simulink model "Model_6DOF_B3"  (R2020b)
settings: Solver=FixedStepAuto  StartTime=0.0  StopTime=120  FixedStep=0.05  RelTol=1e-3
values from neighbouring files (symbols this model uses):
  Ba_0 = [0 0 0 0 0 0]    [ctrl_mode_param.m]
  Bb = 4418825.3321    [load_data.m]
  Bv_0 = [tgt_speed 0 0 0 0 0]    [ctrl_mode_param.m]
  Bx_0 = [0 0 tgt_depth 0 0 0]    [ctrl_mode_param.m]
  Ixx = 5.23e7    (= 52300000)    [load_data.m]
  Ixy = 0    [load_data.m]
  Ixz = 0    [load_data.m]
  Iyy = 1.375e9    (= 1375000000)    [load_data.m]
  Iyz = 0    [load_data.m]
  Izz = 1.367e9    (= 1367000000)    [load_data.m]
  Mb = 4418825.3321    [load_data.m]
  Xb = 0    [load_data.m]
  Xg = 0    [load_data.m]
  Yb = 0    [load_data.m]
  Yg = 0    [load_data.m]
  Zb = 0.4406    [load_data.m]
  Zg = 0    [load_data.m]
undefined symbols (not defined in the file or in its folder): dA_BP1, dA_BP2, dA_Hull, dA_PH, dA_Sail, dA_SProot, dA_X1a, dA_X1b, dA_X2a, dA_X2b, dA_X3a, dA_X3b, dA_X4a, dA_X4b, its, n_BP1, n_BP2, n_Hull, n_PH, n_Sail, n_SProot, n_X1a, n_X1b, n_X2a, n_X2b, n_X3a, n_X3b, n_X4a, n_X4b, nt_BP1, nt_BP2, nt_Hull, nt_PH, nt_Sail, nt_SProot, nt_X1a, nt_X1b, nt_X2a, nt_X2b, nt_X3a, nt_X3b, nt_X4a, nt_X4b, Usp, vt1_BP1, vt1_BP2, vt1_Hull, vt1_PH, vt1_Sail, vt1_SProot, vt1_X1a, vt1_X1b, vt1_X2a, vt1_X2b, vt1_X3a, vt1_X3b, vt1_X4a, vt1_X4b, vt2_BP1, vt2_BP2 ... (+27)
libraries: simulink x5
(part 9 of 15)

== system Model_6DOF_B3/HDM B3/Wave, Virtual Mass and Hydrostatic/Wave Particle Motions ==
  U_ship : Inport
  X_earth : Inport  Port=2
  CGi : Inport  Port=3
  CG : Inport  Port=4
  SeaState : Inport  Port=5
  dLCG : Inport  Port=6
  dX_CTRL : Inport  Port=7
  fwrite : Inport  Port=8
  Add : Sum  Inputs=+-
  Clock : Clock
  Constant : Constant  Value=3
  Constant1 : Constant  Value=Zb
  Constant2 : Constant  Value=0.474
  Constant6 : Constant  Value=1025
  Constant7 : Constant  Value=9.81
  Local eff. Depth : MATLAB Function  TreatAsAtomicUnit=on
  MATLAB Function1 : MATLAB Function  TreatAsAtomicUnit=on
  Mux : Mux  Inputs=5
  Sectional Position Vectors : MATLAB Function  TreatAsAtomicUnit=on
  Sectional Wave Particle & Rigid Body Velocities : MATLAB Function  TreatAsAtomicUnit=on
  Subsystem : Subsystem
  Wave Properties : MATLAB Function  TreatAsAtomicUnit=on
  Wave particle velocity at hull CG : MATLAB Function  TreatAsAtomicUnit=on
  X_SP1 : Constant  Value=[31.924; 3.861; -3.861;]
  X_SP2 : Constant  Value=[31.924; 3.861; 3.861;]
  X_SP3 : Constant  Value=[31.924; -3.861; 3.861;]
  X_SP4 : Constant  Value=[31.924; -3.861; -3.861;]
  X_XB : Constant  Value=[-10.465; 0; 9.732;]
  beta_wave : Constant  Value=0
  phi_wave : Constant  Value=0
  Rs : Outport
  zeff : Outport  Port=2
  uwXis : Outport  Port=3
  uwsCG : Outport  Port=4
  uws : Outport  Port=5
  urs : Outport  Port=6
  B_FM : Outport  Port=7
  wires:
  Sectional Position Vectors/2(Rs) -> Sectional Wave Particle & Rigid Body Velocities/5(Rs), Rs/1
  SeaState/1 -> Wave Properties/1(SeaState)
  Clock/1 -> MATLAB Function1/1(time), Wave particle velocity at hull CG/1(time), Local eff. Depth/1(time), Sectional Wave Particle & Rigid Body Velocities/1(time), Subsystem/1(time)
  Sectional Position Vectors/1(Xce) -> Sectional Wave Particle & Rigid Body Velocities/4(Xce)
  X_earth/1 -> Subsystem/2(Xearth), Sectional Wave Particle & Rigid Body Velocities/3(X_earth), MATLAB Function1/7(X_earth), Wave particle velocity at hull CG/2(X_earth), Local eff. Depth/2(Bxe), Sectional Position Vectors/1(X_earth)
  Wave Properties/3(k_wave) -> Subsystem/4(k_wave), Wave particle velocity at hull CG/8(k_wave), Local eff. Depth/3(k_wave), MATLAB Function1/13(k_wave), Sectional Wave Particle & Rigid Body Velocities/10(k_wave)  "k"
  U_ship/1 -> MATLAB Function1/8(U_ship), Sectional Wave Particle & Rigid Body Velocities/2(U_ship)
  Wave Properties/1(L_wave) -> MATLAB Function1/9(L_wave), Sectional Wave Particle & Rigid Body Velocities/8(L_wave), Wave particle velocity at hull CG/4(L_wave)
  Wave Properties/4(w_wave) -> Subsystem/5(w_wave), Wave particle velocity at hull CG/9(w_wave), Local eff. Depth/4(w_wave), MATLAB Function1/14(w_wave), Sectional Wave Particle & Rigid Body Velocities/11(w_wave)  "w"
  CGi/1 -> Sectional Position Vectors/2(CGi)
  CG/1 -> Sectional Position Vectors/3(CG)
  Sectional Wave Particle & Rigid Body Velocities/2(Urs) -> urs/1
  Sectional Wave Particle & Rigid Body Velocities/1(Uws) -> uws/1
  dLCG/1 -> Wave particle velocity at hull CG/3(dLCG), Sectional Position Vectors/4(dLCG)
  Wave Properties/2(A_wave) -> Subsystem/3(A_wave), Wave particle velocity at hull CG/7(A_wave), Local eff. Depth/5(a_wave), MATLAB Function1/12(A_wave), Sectional Wave Particle & Rigid Body Velocities/9(A_wave)
  Local eff. Depth/1(z_eff) -> zeff/1
  X_XB/1 -> MATLAB Function1/6(rXB)
  X_SP4/1 -> MATLAB Function1/5(rX4)
  X_SP3/1 -> MATLAB Function1/4(rX3)
  X_SP2/1 -> MATLAB Function1/3(rX2)
  X_SP1/1 -> MATLAB Function1/2(rX1)
  MATLAB Function1/1(uwX1s) -> Mux/1
  MATLAB Function1/2(uwX2s) -> Mux/2
  MATLAB Function1/3(uwX3s) -> Mux/3
  MATLAB Function1/4(uwX4s) -> Mux/4
  MATLAB Function1/5(uwXBs) -> Mux/5
  Mux/1 -> uwXis/1
  phi_wave/1 -> Sectional Wave Particle & Rigid Body Velocities/6(phi_wave), Wave particle velocity at hull CG/5(phi_wave), MATLAB Function1/10(phi_wave)
  beta_wave/1 -> MATLAB Function1/11(beta_wave), Sectional Wave Particle & Rigid Body Velocities/7(beta_wave), Wave particle velocity at hull CG/6(beta_wave)
  Wave particle velocity at hull CG/1(uwsCG) -> uwsCG/1
  Constant/1 -> Sectional Wave Particle & Rigid Body Velocities/12(iProbe)
  Subsystem/1(Out1) -> B_FM/1
  Constant6/1 -> Subsystem/6(rho)
  Constant7/1 -> Subsystem/7(g)
  Add/1 -> Subsystem/8(Zb)
  Constant2/1 -> Add/1
  Constant1/1 -> Add/2
  dX_CTRL/1 -> Subsystem/9(dX_CTRL)
  fwrite/1 -> Subsystem/10(fwrite)

== system Model_6DOF_B3/HDM B3/X/X'dXi ==
  UeX : Inport
  dXeff : Inport  Port=2
  Gain : Gain  Gain=-1
  Gain{4..7} (4 alike) : Gain
  Mux : Mux  Inputs=5
  Saturation6 : Saturate  UpperLimit=-1.543332  LowerLimit=-5.14444
  Selector10 : Selector  InputPortWidth=5  IndexOptions=Index vector (dialog)  Indices=4  OutputSizes=1
  Selector11 : Selector  InputPortWidth=5  IndexOptions=Index vector (dialog)  Indices=4  OutputSizes=1
  Selector12 : Selector  InputPortWidth=5  IndexOptions=Index vector (dialog)  Indices=5  OutputSizes=1
  Selector2 : Selector  InputPortWidth=5  IndexOptions=Index vector (dialog)  Indices=5  OutputSizes=1
  Selector4 : Selector  InputPortWidth=5  IndexOptions=Index vector (dialog)  Indices=1  OutputSizes=1
  Selector5 : Selector  InputPortWidth=5  IndexOptions=Index vector (dialog)  Indices=1  OutputSizes=1
  Selector6 : Selector  InputPortWidth=5  IndexOptions=Index vector (dialog)  Indices=2  OutputSizes=1
  Selector7 : Selector  InputPortWidth=5  IndexOptions=Index vector (dialog)  Indices=2  OutputSizes=1
  Selector8 : Selector  InputPortWidth=5  IndexOptions=Index vector (dialog)  Indices=3  OutputSizes=1
  Selector9 : Selector  InputPortWidth=5  IndexOptions=Index vector (dialog)  Indices=3  OutputSizes=1
  To Workspace : ToWorkspace  VariableName=UeX  SaveFormat=Timeseries  SampleTime=-1
  XudX1 : Lookup_n-D  BreakpointsForDimension1=[-30 -20 -10 0 10 20 30]  BreakpointsForDimension2=|  Table=|  InternalRulePriority=Speed  RndMeth=Simplest  InputSameDT=on
      BreakpointsForDimension2=|
      | [-7.716666
      | -5.144444
      | -3.0866664
      | -1.5433332
      | ]
      Table=|
      | reshape([3.2151E-04
      | 1.4055E-04
      | 2.3723E-05
      | -2.9685E-05
      | 2.3777E-05
      | 1.3375E-04
      | 3.3722E-04
      | 1.6076E-04
      | 7.0275E-05
      | 1.1862E-05
      | -1.4843E-05
      | 1.1889E-05
      | 6.6875E-05
      | 1.6861E-04
      | 1.6698E-04
      | 6.8790E-05
      | 1.2322E-05
      | -1.4312E-05
      | 1.2274E-05
      | 6.7265E-05
      | 1.7083E-04
      | 3.4224E-04
      | 1.3333E-04
      | 2.5937E-05
      | -6.5668E-05
      | 2.5937E-05
      | 1.3102E-04
      | 3.4214E-04
      | ],[7,4])
      settings: InputPortMap=u0,u1
  XudX2 : Lookup_n-D  BreakpointsForDimension1=[-30 -20 -10 0 10 20 30]  BreakpointsForDimension2=|  Table=|  InternalRulePriority=Speed  RndMeth=Simplest  InputSameDT=on
      BreakpointsForDimension2=|
      | [-7.716666
      | -5.144444
      | -3.0866664
      | -1.5433332
      | ]
      Table=|
      | reshape([2.9233E-04
      | 1.3189E-04
      | 2.3224E-05
      | -2.9022E-05
      | 1.9675E-05
      | 1.4726E-04
      | 3.7676E-04
      | 1.4617E-04
      | 6.5945E-05
      | 1.1612E-05
      | -1.4511E-05
      | 9.8375E-06
      | 7.3630E-05
      | 1.8838E-04
      | 1.7319E-04
      | 6.7285E-05
      | 1.2060E-05
      | -2.5958E-05
      | 1.0337E-05
      | 7.6660E-05
      | 1.8963E-04
      | 3.4748E-04
      | 1.3335E-04
      | 2.2395E-05
      | -2.6403E-05
      | 2.2395E-05
      | 1.5181E-04
      | 3.8598E-04
      | ],[7,4])
      settings: InputPortMap=u0,u1
  XudX3 : Lookup_n-D  BreakpointsForDimension1=[-30 -20 -10 0 10 20 30]  BreakpointsForDimension2=|  Table=|  InternalRulePriority=Speed  RndMeth=Simplest  InputSameDT=on
      BreakpointsForDimension2=|
      | [-7.716666
      | -5.144444
      | -3.0866664
      | -1.5433332
      | ]
      Table=|
      | reshape([3.5642E-04
      | 1.5674E-04
      | 2.5449E-05
      | -2.9060E-05
      | 2.6726E-05
      | 1.6225E-04
      | 3.1115E-04
      | 1.7821E-04
      | 7.8370E-05
      | 1.2725E-05
      | -1.4530E-05
      | 1.3363E-05
      | 8.1125E-05
      | 1.5558E-04
      | 1.9053E-04
      | 8.0600E-05
      | 1.2911E-05
      | -1.3998E-05
      | 1.3672E-05
      | 7.4645E-05
      | 1.6290E-04
      | 3.8447E-04
      | 1.4526E-04
      | 2.7824E-05
      | -2.6434E-05
      | 2.7824E-05
      | 1.5039E-04
      | 3.2499E-04
      | ],[7,4])
      settings: InputPortMap=u0,u1
  XudX4 : Lookup_n-D  BreakpointsForDimension1=[-30 -20 -10 0 10 20 30]  BreakpointsForDimension2=|  Table=|  InternalRulePriority=Speed  RndMeth=Simplest  InputSameDT=on
      BreakpointsForDimension2=|
      | [-7.716666
      | -5.144444
      | -3.0866664
      | -1.5433332
      | ]
      Table=|
      | reshape([3.4525E-04
      | 1.3840E-04
      | 2.4668E-05
      | -2.9702E-05
      | 2.4205E-05
      | 1.2737E-04
      | 3.2790E-04
      | 1.7263E-04
      | 6.9200E-05
      | 1.2334E-05
      | -1.4851E-05
      | 1.2103E-05
      | 6.3685E-05
      | 1.6395E-04
      | 1.7298E-04
      | 6.9435E-05
      | 1.2696E-05
      | -1.4315E-05
      | 1.2608E-05
      | 6.9175E-05
      | 1.6779E-04
      | 3.3803E-04
      | 1.5513E-04
      | 2.6677E-05
      | -2.7052E-05
      | 2.6677E-05
      | 1.3644E-04
      | 3.3780E-04
      | ],[7,4])
      settings: InputPortMap=u0,u1
  XudXB : Lookup_n-D  BreakpointsForDimension1=[-30 -20 -10 0 10 20 30]  BreakpointsForDimension2=[-5.14444 -3.08666664 -1.54332]  Table=|  InternalRulePriority=Speed  RndMeth=Simplest  InputSameDT=on
      | reshape([6.9060E-04
      | 3.9256E-04
      | 1.5651E-04
      | 0.0000E+00
      | 1.1449E-04
      | 4.2412E-04
      | 5.7370E-04
      | 6.4542E-04
      | 3.9138E-04
      | 1.5593E-04
      | 0.0000E+00
      | 1.1381E-04
      | 4.1205E-04
      | 5.6813E-04
      | 6.5675E-04
      | 3.9410E-04
      | 1.1271E-04
      | 0.0000E+00
      | 1.1271E-04
      | 4.2649E-04
      | 5.7604E-04
      | ],[7,3])
      settings: InputPortMap=u0,u1
  Out1 : Outport
  wires:
  Selector2/1 -> XudXB/1
  XudX4/1 -> Gain7/1
  XudX3/1 -> Gain5/1
  XudX2/1 -> Gain6/1
  XudX1/1 -> Gain4/1
  Mux/1 -> Out1/1
  dXeff/1 -> Selector2/1, Selector10/1, Selector8/1, Selector6/1, Selector4/1
  Selector4/1 -> XudX1/1
  Selector5/1 -> XudX1/2
  Selector6/1 -> XudX2/1
  Selector7/1 -> XudX2/2
  Selector8/1 -> XudX3/1
  Selector9/1 -> XudX3/2
  UeX/1 -> Gain/1
  Selector11/1 -> XudX4/2
  Selector10/1 -> XudX4/1
  Selector12/1 -> XudXB/2
  Gain4/1 -> Mux/1
  Gain6/1 -> Mux/2
  Gain5/1 -> Mux/3
  Gain7/1 -> Mux/4
  XudXB/1 -> Mux/5
  Gain/1 -> To Workspace/1, Saturation6/1
  Saturation6/1 -> Selector11/1, Selector12/1, Selector9/1, Selector7/1, Selector5/1

== system Model_6DOF_B3/HDM B3/X 6d org/Subsystem1 ==
  UeX : Inport
  dXeff : Inport  Port=2
  z : Inport  Port=3
  Demux : Demux  Outputs=5
  Demux1 : Demux  Outputs=5
  Mux : Mux  Inputs=5
  Xud4 : Lookup_n-D  NumberOfTableDimensions=3  BreakpointsForDimension1=[-30 -20 -10 0 10 20 30]  BreakpointsForDimension2=|  BreakpointsForDimension3=|  Table=|  InternalRulePriority=Speed  RndMeth=Simplest  InputSameDT=on
      BreakpointsForDimension2=|
      | [1.5433332
      | 3.0866664
      | 
      | 5.144444]
      BreakpointsForDimension3=|
      | [-36.3724
      | -18.3724
      | -15.3724
      | -13.8724]
      Table=|
      | reshape([1.9515E-04
      | 1.0370E-04
      | 3.9468E-05
      | 1.2612E-05
      | 3.9477E-05
      | 9.2497E-05
      | 1.9504E-04
      | 2.0037E-04
      | 9.3994E-05
      | 3.9650E-05
      | 1.2608E-05
      | 3.9217E-05
      | 9.5451E-05
      | 1.8893E-04
      | 2.0342E-04
      | 9.8349E-05
      | 3.9739E-05
      | 1.2608E-05
      | 3.9126E-05
      | 9.3002E-05
      | 1.9310E-04
      | 2.0342E-04
      | 9.7784E-05
      | 3.9737E-05
      | 1.2594E-05
      | 3.8955E-05
      | 9.3472E-05
      | 1.8818E-04
      | 1.9912E-04
      | 9.6216E-05
      | 3.8834E-05
      | 1.1823E-05
      | 3.8745E-05
      | 9.5316E-05
      | 1.9299E-04
      | 2.0055E-04
      | 9.7244E-05
      | 3.9050E-05
      | 1.1812E-05
      | 3.8434E-05
      | 9.0497E-05
      | 1.8966E-04
      | 2.6693E-04
      | 1.4022E-04
      | 3.8561E-05
      | 1.1822E-05
      | 3.3455E-05
      | 1.0520E-04
      | 2.4359E-04
      | 2.0044E-04
      | 1.0295E-04
      | 3.9158E-05
      | 1.1774E-05
      | 3.8178E-05
      | 9.0714E-05
      | 1.8818E-04
      | 1.9655E-04
      | 9.5339E-05
      | 3.8472E-05
      | 1.1287E-05
      | 3.8241E-05
      | 9.3683E-05
      | 1.8812E-04
      | 1.9890E-04
      | 9.7584E-05
      | 3.8662E-05
      | 1.1263E-05
      | 3.7865E-05
      | 8.8045E-05
      | 1.8986E-04
      | 2.6693E-04
      | 1.4022E-04
      | 3.8561E-05
      | 1.1263E-05
      | 3.3455E-05
      | 1.0520E-04
      | 2.4359E-04
      | 2.0199E-04
      | 9.6354E-05
      | 3.8835E-05
      | 1.1203E-05
      | 3.7555E-05
      | 8.7551E-05
      | 1.8761E-04],[7,3,4])
      settings: InputPortMap=u0,u1,u2
  XudX1 : Lookup_n-D  NumberOfTableDimensions=3  BreakpointsForDimension1=[-30 -20 -10 0 10 20 30]  BreakpointsForDimension2=|  BreakpointsForDimension3=|  Table=|  InternalRulePriority=Speed  RndMeth=Simplest  InputSameDT=on
      BreakpointsForDimension2=|
      | [1.5433332
      | 3.0866664
      | 
      | 5.144444]
      BreakpointsForDimension3=|
      | [-36.3724
      | -18.3724
      | -15.3724
      | -13.8724]
      Table=|
      | reshape([1.9726E-04
      | 9.2807E-05
      | 3.9153E-05
      | 1.2612E-05
      | 3.9108E-05
      | 9.6157E-05
      | 1.9721E-04
      | 1.9513E-04
      | 9.5505E-05
      | 3.8964E-05
      | 1.2607E-05
      | 3.9329E-05
      | 9.6357E-05
      | 1.9540E-04
      | 1.9473E-04
      | 1.0389E-04
      | 3.8933E-05
      | 1.2607E-05
      | 3.9448E-05
      | 9.9420E-05
      | 2.0231E-04
      | 1.9473E-04
      | 1.0019E-04
      | 3.8828E-05
      | 1.2592E-05
      | 3.9441E-05
      | 9.3211E-05
      | 2.0035E-04
      | 1.9312E-04
      | 9.4955E-05
      | 3.8460E-05
      | 1.1826E-05
      | 3.8411E-05
      | 9.3406E-05
      | 1.9672E-04
      | 1.9062E-04
      | 9.2834E-05
      | 3.8250E-05
      | 1.1814E-05
      | 3.8668E-05
      | 9.2911E-05
      | 1.9753E-04
      | 2.4353E-04
      | 1.0500E-04
      | 3.3326E-05
      | 1.1821E-05
      | 3.8282E-05
      | 1.3081E-04
      | 2.5995E-04
      | 1.8933E-04
      | 9.3556E-05
      | 3.8050E-05
      | 1.1773E-05
      | 3.8871E-05
      | 9.3887E-05
      | 2.0035E-04
      | 1.8690E-04
      | 9.6416E-05
      | 3.7999E-05
      | 1.1295E-05
      | 3.8027E-05
      | 9.1995E-05
      | 1.9449E-04
      | 1.9009E-04
      | 9.2479E-05
      | 3.7675E-05
      | 1.1269E-05
      | 3.8335E-05
      | 8.9889E-05
      | 1.9665E-04
      | 2.4353E-04
      | 1.0500E-04
      | 3.3326E-05
      | 1.1269E-05
      | 3.8282E-05
      | 1.3081E-04
      | 2.5995E-04
      | 1.8646E-04
      | 9.1163E-05
      | 3.7419E-05
      | 1.1206E-05
      | 3.8643E-05
      | 9.8736E-05
      | 2.0514E-04],[7,3,4])
      settings: InputPortMap=u0,u1,u2
  XudX1B : Lookup_n-D  NumberOfTableDimensions=3  BreakpointsForDimension1=[-30 -20 -10 0 10 20 30]  BreakpointsForDimension2=|  BreakpointsForDimension3=|  Table=|  InternalRulePriority=Speed  RndMeth=Simplest  InputSameDT=on
      BreakpointsForDimension2=|
      | [1.5433332
      | 3.0866664
      | 
      | 5.144444]
      BreakpointsForDimension3=|
      | [-36.3724
      | -18.3724
      | -15.3724
      | -13.8724]
      Table=|
      | reshape([3.9535E-04
      | 2.6403E-04
      | 1.4465E-04
      | 6.6976E-05
      | 1.2333E-04
      | 2.8515E-04
      | 3.5499E-04
      | 3.8973E-04
      | 2.6514E-04
      | 1.4731E-04
      | 6.8622E-05
      | 1.2628E-04
      | 2.9201E-04
      | 3.6632E-04
      | 4.0285E-04
      | 2.7250E-04
      | 1.4933E-04
      | 6.8622E-05
      | 1.2952E-04
      | 2.9373E-04
      | 3.6588E-04
      | 4.0285E-04
      | 2.8332E-04
      | 1.5162E-04
      | 7.2213E-05
      | 1.3467E-04
      | 3.0293E-04
      | 3.6349E-04
      | 3.8950E-04
      | 2.6292E-04
      | 1.4475E-04
      | 6.6785E-05
      | 1.2369E-04
      | 2.7281E-04
      | 3.4895E-04
      | 3.9519E-04
      | 2.6529E-04
      | 1.4760E-04
      | 6.8542E-05
      | 1.2717E-04
      | 2.7841E-04
      | 3.6301E-04
      | 5.6904E-04
      | 3.2107E-04
      | 1.3512E-04
      | 7.0542E-05
      | 1.0919E-04
      | 4.1259E-04
      | 6.2735E-04
      | 3.6838E-04
      | 3.0195E-04
      | 1.5438E-04
      | 7.4592E-05
      | 1.4048E-04
      | 3.1396E-04
      | 3.6349E-04
      | 4.1126E-04
      | 2.6224E-04
      | 1.4422E-04
      | 6.5961E-05
      | 1.2321E-04
      | 2.7802E-04
      | 3.5744E-04
      | 4.0057E-04
      | 2.6952E-04
      | 1.4782E-04
      | 6.8341E-05
      | 1.2789E-04
      | 2.8978E-04
      | 3.5944E-04
      | 5.6904E-04
      | 3.2107E-04
      | 1.3512E-04
      | 6.8341E-05
      | 1.0919E-04
      | 4.1259E-04
      | 6.2735E-04
      | 4.8319E-04
      | 3.1751E-04
      | 1.5761E-04
      | 7.4804E-05
      | 1.3557E-04
      | 3.2741E-04
      | 4.7146E-04],[7,3,4])
      settings: InputPortMap=u0,u1,u2
  XudX2 : Lookup_n-D  NumberOfTableDimensions=3  BreakpointsForDimension1=[-30 -20 -10 0 10 20 30]  BreakpointsForDimension2=|  BreakpointsForDimension3=|  Table=|  InternalRulePriority=Speed  RndMeth=Simplest  InputSameDT=on
      BreakpointsForDimension2=|
      | [1.5433332
      | 3.0866664
      | 
      | 5.144444]
      BreakpointsForDimension3=|
      | [-36.3724
      | -18.3724
      | -15.3724
      | -13.8724]
      Table=|
      | reshape([1.9988E-04
      | 9.2815E-05
      | 3.8984E-05
      | 1.2936E-05
      | 3.7333E-05
      | 1.0938E-04
      | 2.1913E-04
      | 2.0000E-04
      | 9.3101E-05
      | 3.8429E-05
      | 1.2739E-05
      | 3.7583E-05
      | 1.1064E-04
      | 2.1950E-04
      | 2.0083E-04
      | 9.4269E-05
      | 3.8054E-05
      | 1.2739E-05
      | 3.7662E-05
      | 1.0858E-04
      | 2.2083E-04
      | 2.0083E-04
      | 9.5605E-05
      | 3.7864E-05
      | 1.2538E-05
      | 3.7776E-05
      | 1.1595E-04
      | 2.1404E-04
      | 1.9933E-04
      | 9.2999E-05
      | 3.8198E-05
      | 1.2159E-05
      | 3.6475E-05
      | 1.0280E-04
      | 2.1737E-04
      | 2.0006E-04
      | 9.3307E-05
      | 3.7549E-05
      | 1.1957E-05
      | 3.6899E-05
      | 1.1530E-04
      | 2.2066E-04
      | 2.4216E-04
      | 1.0448E-04
      | 2.9342E-05
      | 1.1821E-05
      | 3.5012E-05
      | 1.3098E-04
      | 2.3359E-04
      | 1.9082E-04
      | 9.0828E-05
      | 3.6826E-05
      | 1.1709E-05
      | 3.7301E-05
      | 1.0927E-04
      | 2.1404E-04
      | 1.6701E-04
      | 9.2083E-05
      | 3.7750E-05
      | 1.1627E-05
      | 3.5975E-05
      | 9.9381E-05
      | 2.1803E-04
      | 1.9264E-04
      | 9.0003E-05
      | 3.6917E-05
      | 1.1397E-05
      | 3.6539E-05
      | 1.0523E-04
      | 2.1540E-04
      | 2.4216E-04
      | 1.0448E-04
      | 2.9342E-05
      | 1.1397E-05
      | 3.5012E-05
      | 1.3098E-04
      | 2.3359E-04
      | 1.8911E-04
      | 9.0019E-05
      | 3.6083E-05
      | 1.1213E-05
      | 3.7708E-05
      | 1.0882E-04
      | 1.6878E-04],[7,3,4])
      settings: InputPortMap=u0,u1,u2
  XudX3 : Lookup_n-D  NumberOfTableDimensions=3  BreakpointsForDimension1=[-30 -20 -10 0 10 20 30]  BreakpointsForDimension2=|  BreakpointsForDimension3=|  Table=|  InternalRulePriority=Speed  RndMeth=Simplest  InputSameDT=on
      BreakpointsForDimension2=|
      | [1.5433332
      | 3.0866664
      | 
      | 5.144444]
      BreakpointsForDimension3=|
      | [-36.3724
      | -18.3724
      | -15.3724
      | -13.8724]
      Table=|
      | reshape([2.1838E-04
      | 9.8768E-05
      | 3.9298E-05
      | 1.2921E-05
      | 4.0048E-05
      | 1.0549E-04
      | 1.8864E-04
      | 2.2881E-04
      | 1.0336E-04
      | 3.9060E-05
      | 1.2736E-05
      | 3.9535E-05
      | 1.0325E-04
      | 1.9538E-04
      | 2.1692E-04
      | 1.0227E-04
      | 3.8885E-05
      | 1.2736E-05
      | 3.9285E-05
      | 9.9666E-05
      | 1.9406E-04
      | 2.1692E-04
      | 1.0151E-04
      | 3.8619E-05
      | 1.2552E-05
      | 3.9212E-05
      | 1.0291E-04
      | 2.0160E-04
      | 2.1667E-04
      | 1.0323E-04
      | 3.9049E-05
      | 1.2140E-05
      | 3.9810E-05
      | 1.0079E-04
      | 1.9039E-04
      | 2.2496E-04
      | 9.9708E-05
      | 3.8786E-05
      | 1.1948E-05
      | 3.9280E-05
      | 1.0040E-04
      | 1.8622E-04
      | 2.7315E-04
      | 1.3714E-04
      | 3.4983E-05
      | 1.1821E-05
      | 3.1018E-05
      | 1.0427E-04
      | 1.9674E-04
      | 2.2211E-04
      | 1.0444E-04
      | 3.8528E-05
      | 1.1713E-05
      | 3.8636E-05
      | 9.5401E-05
      | 2.0160E-04
      | 2.0348E-04
      | 1.0451E-04
      | 3.8863E-05
      | 1.1608E-05
      | 3.9501E-05
      | 1.0479E-04
      | 1.8840E-04
      | 2.0541E-04
      | 9.7216E-05
      | 3.8561E-05
      | 1.1388E-05
      | 3.8824E-05
      | 9.5169E-05
      | 1.8576E-04
      | 2.7315E-04
      | 1.3714E-04
      | 3.4983E-05
      | 1.1388E-05
      | 3.1018E-05
      | 1.0427E-04
      | 1.9674E-04
      | 2.1961E-04
      | 1.1536E-04
      | 3.8716E-05
      | 1.1221E-05
      | 3.7813E-05
      | 9.5976E-05
      | 1.9612E-04],[7,3,4])
      settings: InputPortMap=u0,u1,u2
  XdXi : Outport
  wires:
  Mux/1 -> XdXi/1
  XudX1/1 -> Mux/1
  XudX2/1 -> Mux/2
  Xud4/1 -> Mux/4
  dXeff/1 -> Demux1/1
  UeX/1 -> Demux/1
  XudX3/1 -> Mux/3
  XudX1B/1 -> Mux/5
  Demux/1 -> XudX1/2
  Demux/2 -> XudX2/2
  Demux/3 -> XudX3/2
  Demux/4 -> Xud4/2
  Demux/5 -> XudX1B/2
  z/1 -> XudX1/3, XudX2/3, XudX3/3, XudX1B/3, Xud4/3
  Demux1/1 -> XudX1/1
  Demux1/2 -> XudX2/1
  Demux1/3 -> XudX3/1
  Demux1/5 -> XudX1B/1
  Demux1/4 -> Xud4/1

== system Model_6DOF_B3/HDM B3/Y/YdXi ==
  dX : Inport
  z : Inport  Port=2
  Mux : Mux
  Selector1 : Selector  InputPortWidth=5  IndexOptions=Index vector (dialog)  Indices=2  OutputSizes=1
  Selector2 : Selector  InputPortWidth=5  IndexOptions=Index vector (dialog)  Indices=3  OutputSizes=1
  Selector3 : Selector  InputPortWidth=5  IndexOptions=Index vector (dialog)  Indices=4  OutputSizes=1
  Selector7 : Selector  InputPortWidth=5  IndexOptions=Index vector (dialog)  Indices=1  OutputSizes=1
  YdX1 : Lookup_n-D  BreakpointsForDimension1=[-10 0 10]  BreakpointsForDimension2=|  BreakpointsForDimension3=[-5.14444 -3.08666664 -1.54332]  Table=|  InternalRulePriority=Speed  RndMeth=Simplest  InputSameDT=on
      BreakpointsForDimension2=|
      | [-36.4062987
      | -18.4062987
      | -15.4062987
      | -13.9062987]
      Table=|
      | reshape([-1.8282E-04
      | -6.0037E-06
      | 1.6496E-04
      | -1.7978E-04
      | -2.4314E-06
      | 1.6969E-04
      | -1.4480E-04
      | -2.4314E-06
      | 2.0267E-04
      | -1.7641E-04
      | 1.4850E-06
      | 1.7514E-04],[3,4])
      settings: InputPortMap=u0,u1
  YdX2 : Lookup_n-D  BreakpointsForDimension1=[-10 0 10]  BreakpointsForDimension2=|  BreakpointsForDimension3=[-5.14444 -3.08666664 -1.54332]  Table=|  InternalRulePriority=Speed  RndMeth=Simplest  InputSameDT=on
      BreakpointsForDimension2=|
      | [-36.4062987
      | -18.4062987
      | -15.4062987
      | -13.9062987]
      Table=|
      | reshape([1.4857E-04
      | -6.6611E-06
      | -1.5932E-04
      | 1.4200E-04
      | -1.2968E-05
      | -1.6860E-04
      | 9.4982E-05
      | -1.2968E-05
      | -2.1344E-04
      | 1.3366E-04
      | -2.3176E-05
      | -1.8599E-04],[3,4])
      settings: InputPortMap=u0,u1
  YdX3 : Lookup_n-D  BreakpointsForDimension1=[-10 0 10]  BreakpointsForDimension2=|  BreakpointsForDimension3=[-5.14444 -3.08666664 -1.54332]  Table=|  InternalRulePriority=Speed  RndMeth=Simplest  InputSameDT=on
      BreakpointsForDimension2=|
      | [-36.4062987
      | -18.4062987
      | -15.4062987
      | -13.9062987]
      Table=|
      | reshape([2.0207E-04
      | 6.9701E-06
      | -1.9141E-04
      | 2.0588E-04
      | 1.3213E-05
      | -1.8007E-04
      | 2.2753E-04
      | 1.3213E-05
      | -1.0937E-04
      | 2.1222E-04
      | 2.3270E-05
      | -1.6161E-04],[3,4])
      settings: InputPortMap=u0,u1
  YdX4 : Lookup_n-D  BreakpointsForDimension1=[-10 0 10]  BreakpointsForDimension2=|  BreakpointsForDimension3=[-5.14444 -3.08666664 -1.54332]  Table=|  InternalRulePriority=Speed  RndMeth=Simplest  InputSameDT=on
      BreakpointsForDimension2=|
      | [-36.4062987
      | -18.4062987
      | -15.4062987
      | -13.9062987]
      Table=|
      | reshape([-1.7022E-04
      | 5.9932E-06
      | 1.8722E-04
      | -1.7390E-04
      | 2.3770E-06
      | 1.8293E-04
      | -2.0489E-04
      | 2.3770E-06
      | 1.4658E-04
      | -1.7771E-04
      | -1.6689E-06
      | 1.7805E-04],[3,4])
      settings: InputPortMap=u0,u1
  YdX : Outport
  wires:
  Mux/1 -> YdX/1
  z/1 -> YdX4/2, YdX3/2, YdX2/2, YdX1/2
  YdX1/1 -> Mux/1
  YdX2/1 -> Mux/2
  YdX3/1 -> Mux/3
  YdX4/1 -> Mux/4
  Selector7/1 -> YdX1/1
  dX/1 -> Selector2/1, Selector3/1, Selector1/1, Selector7/1
  Selector3/1 -> YdX4/1
  Selector2/1 -> YdX3/1
  Selector1/1 -> YdX2/1

== system Model_6DOF_B3/HDM B3/Z/ZdXi ==
  dX : Inport
  z : Inport  Port=2
  Demux6 : Demux  Outputs=5
  Mux : Mux  Inputs=5
  ZudX1 q+10 : Lookup_n-D  BreakpointsForDimension1=[-30 -20 -10 0 10 20 30]  BreakpointsForDimension2=[-35.0624 -15.3724 -13.8724]  BreakpointsForDimension3=[-35.0624 -15.3724 -13.8724]  Table=|  InternalRulePriority=Speed  RndMeth=Simplest  InputSameDT=on
      | reshape([-0.003226964
      | -0.002116041
      | -0.001005119
      | 0.000105803
      | 0.001216725
      | 0.002327647
      | 0.003438569
      | -0.003036597
      | -0.001876165
      | -0.000715732
      | 0.0004447
      | 0.001605132
      | 0.002765565
      | 0.003925997
      | -0.003676642
      | -0.002490275
      | -0.001303908
      | -0.000117541
      | 0.001068826
      | 0.002255193
      | 0.00344156],[7,3])
      settings: InputPortMap=u0,u1
  ZudX1 q+6 : Lookup_n-D  BreakpointsForDimension1=[-30 -20 -10 0 10 20 30]  BreakpointsForDimension2=[-35.0624 -15.3724 -13.8724]  BreakpointsForDimension3=[-5.14444 -3.08666664 -1.54332]  Table=|  InternalRulePriority=Speed  RndMeth=Simplest  InputSameDT=on
      | reshape([-0.001383757
      | -0.000911
      | -0.000438243
      | 3.45135E-05
      | 0.00050727
      | 0.000980027
      | 0.001452784
      | -0.001383757
      | -0.000911
      | -0.000438243
      | 3.45135E-05
      | 0.00050727
      | 0.000980027
      | 0.001452784
      | -0.001353354
      | -0.000887631
      | -0.000421908
      | 4.38143E-05
      | 0.000509537
      | 0.00097526
      | 0.001440982],[7,3])
      settings: InputPortMap=u0,u1
  ZudX1 q+7 : Lookup_n-D  BreakpointsForDimension1=[-30 -20 -10 0 10 20 30]  BreakpointsForDimension2=[-35.0624 -15.3724 -13.8724]  BreakpointsForDimension3=[-5.14444 -3.08666664 -1.54332]  Table=|  InternalRulePriority=Speed  RndMeth=Simplest  InputSameDT=on
      | reshape([-0.001358511
      | -0.00091651
      | -0.000474508
      | -3.25062E-05
      | 0.000409495
      | 0.000851497
      | 0.001293499
      | -0.001303275
      | -0.00086798
      | -0.000432686
      | 2.60877E-06
      | 0.000437903
      | 0.000873198
      | 0.001308493
      | -0.001263287
      | -0.000836064
      | -0.00040884
      | 1.83841E-05
      | 0.000445608
      | 0.000872832
      | 0.001300056],[7,3])
      settings: InputPortMap=u0,u1
  ZudX1 q+8 : Lookup_n-D  BreakpointsForDimension1=[-30 -20 -10 0 10 20 30]  BreakpointsForDimension2=[-35.0624 -15.3724 -13.8724]  BreakpointsForDimension3=[-5.14444 -3.08666664 -1.54332]  Table=|  InternalRulePriority=Speed  RndMeth=Simplest  InputSameDT=on
      | reshape([0.001309084
      | 0.000864124
      | 0.000419163
      | -2.5798E-05
      | -0.000470759
      | -0.000915719
      | -0.00136068
      | 0.001321953
      | 0.000882434
      | 0.000442915
      | 3.39516E-06
      | -0.000436124
      | -0.000875644
      | -0.001315163
      | 0.001313186
      | 0.000881448
      | 0.000449709
      | 1.79712E-05
      | -0.000413767
      | -0.000845505
      | -0.001277243],[7,3])
      settings: InputPortMap=u0,u1
  ZudX1 q+9 : Lookup_n-D  BreakpointsForDimension1=[-30 -20 -10 0 10 20 30]  BreakpointsForDimension2=[-35.0624 -15.3724 -13.8724]  BreakpointsForDimension3=[-5.14444 -3.08666664 -1.54332]  Table=|  InternalRulePriority=Speed  RndMeth=Simplest  InputSameDT=on
      | reshape([0.001464336
      | 0.000977857
      | 0.000491377
      | 4.89775E-06
      | -0.000481582
      | -0.000968061
      | -0.00145454
      | 0.001455937
      | 0.00098192
      | 0.000507903
      | 3.38863E-05
      | -0.00044013
      | -0.000914147
      | -0.001388164
      | 0.001460604
      | 0.00098818
      | 0.000515756
      | 4.33325E-05
      | -0.000429091
      | -0.000901515
      | -0.001373939],[7,3])
      settings: InputPortMap=u0,u1
  ZdX : Outport
  wires:
  ZudX1 q+9/1 -> Mux/4
  ZudX1 q+8/1 -> Mux/3
  ZudX1 q+7/1 -> Mux/2
  ZudX1 q+6/1 -> Mux/1
  ZudX1 q+10/1 -> Mux/5
  z/1 -> ZudX1 q+9/2, ZudX1 q+10/2, ZudX1 q+8/2, ZudX1 q+7/2, ZudX1 q+6/2
  Demux6/5 -> ZudX1 q+10/1
  Mux/1 -> ZdX/1
  Demux6/1 -> ZudX1 q+6/1
  Demux6/2 -> ZudX1 q+7/1
  Demux6/4 -> ZudX1 q+9/1
  dX/1 -> Demux6/1
  Demux6/3 -> ZudX1 q+8/1

== system Model_6DOF_B3/HDM B3/Z 6d org/ZdXi ==
  dX : Inport
  z : Inport  Port=2
  Demux6 : Demux  Outputs=5
  Mux : Mux  Inputs=5
  ZudX1 q+10 : Lookup_n-D  BreakpointsForDimension1=[-30 -20 -10 0 10 20 30]  BreakpointsForDimension2=[-35.0624 -15.3724 -13.8724]  BreakpointsForDimension3=[-35.0624 -15.3724 -13.8724]  Table=|  InternalRulePriority=Speed  RndMeth=Simplest  InputSameDT=on
      | reshape([-0.003226964
      | -0.002116041
      | -0.001005119
      | 0.000105803
      | 0.001216725
      | 0.002327647
      | 0.003438569
      | -0.003036597
      | -0.001876165
      | -0.000715732
      | 0.0004447
      | 0.001605132
      | 0.002765565
      | 0.003925997
      | -0.003676642
      | -0.002490275
      | -0.001303908
      | -0.000117541
      | 0.001068826
      | 0.002255193
      | 0.00344156],[7,3])
      settings: InputPortMap=u0,u1
  ZudX1 q+6 : Lookup_n-D  BreakpointsForDimension1=[-30 -20 -10 0 10 20 30]  BreakpointsForDimension2=[-35.0624 -15.3724 -13.8724]  BreakpointsForDimension3=[-5.14444 -3.08666664 -1.54332]  Table=|  InternalRulePriority=Speed  RndMeth=Simplest  InputSameDT=on
      | reshape([-0.001383757
      | -0.000911
      | -0.000438243
      | 3.45135E-05
      | 0.00050727
      | 0.000980027
      | 0.001452784
      | -0.001383757
      | -0.000911
      | -0.000438243
      | 3.45135E-05
      | 0.00050727
      | 0.000980027
      | 0.001452784
      | -0.001353354
      | -0.000887631
      | -0.000421908
      | 4.38143E-05
      | 0.000509537
      | 0.00097526
      | 0.001440982],[7,3])
      settings: InputPortMap=u0,u1
  ZudX1 q+7 : Lookup_n-D  BreakpointsForDimension1=[-30 -20 -10 0 10 20 30]  BreakpointsForDimension2=[-35.0624 -15.3724 -13.8724]  BreakpointsForDimension3=[-5.14444 -3.08666664 -1.54332]  Table=|  InternalRulePriority=Speed  RndMeth=Simplest  InputSameDT=on
      | reshape([-0.001358511
      | -0.00091651
      | -0.000474508
      | -3.25062E-05
      | 0.000409495
      | 0.000851497
      | 0.001293499
      | -0.001303275
      | -0.00086798
      | -0.000432686
      | 2.60877E-06
      | 0.000437903
      | 0.000873198
      | 0.001308493
      | -0.001263287
      | -0.000836064
      | -0.00040884
      | 1.83841E-05
      | 0.000445608
      | 0.000872832
      | 0.001300056],[7,3])
      settings: InputPortMap=u0,u1
  ZudX1 q+8 : Lookup_n-D  BreakpointsForDimension1=[-30 -20 -10 0 10 20 30]  BreakpointsForDimension2=[-35.0624 -15.3724 -13.8724]  BreakpointsForDimension3=[-5.14444 -3.08666664 -1.54332]  Table=|  InternalRulePriority=Speed  RndMeth=Simplest  InputSameDT=on
      | reshape([0.001309084
      | 0.000864124
      | 0.000419163
      | -2.5798E-05
      | -0.000470759
      | -0.000915719
      | -0.00136068
      | 0.001321953
      | 0.000882434
      | 0.000442915
      | 3.39516E-06
      | -0.000436124
      | -0.000875644
      | -0.001315163
      | 0.001313186
      | 0.000881448
      | 0.000449709
      | 1.79712E-05
      | -0.000413767
      | -0.000845505
      | -0.001277243],[7,3])
      settings: InputPortMap=u0,u1
  ZudX1 q+9 : Lookup_n-D  BreakpointsForDimension1=[-30 -20 -10 0 10 20 30]  BreakpointsForDimension2=[-35.0624 -15.3724 -13.8724]  BreakpointsForDimension3=[-5.14444 -3.08666664 -1.54332]  Table=|  InternalRulePriority=Speed  RndMeth=Simplest  InputSameDT=on
      | reshape([0.001464336
      | 0.000977857
      | 0.000491377
      | 4.89775E-06
      | -0.000481582
      | -0.000968061
      | -0.00145454
      | 0.001455937
      | 0.00098192
      | 0.000507903
      | 3.38863E-05
      | -0.00044013
      | -0.000914147
      | -0.001388164
      | 0.001460604
      | 0.00098818
      | 0.000515756
      | 4.33325E-05
      | -0.000429091
      | -0.000901515
      | -0.001373939],[7,3])
      settings: InputPortMap=u0,u1
  ZdX : Outport
  wires:
  Demux6/3 -> ZudX1 q+8/1
  dX/1 -> Demux6/1
  Demux6/4 -> ZudX1 q+9/1
  Demux6/2 -> ZudX1 q+7/1
  Demux6/1 -> ZudX1 q+6/1
  Demux6/5 -> ZudX1 q+10/1
  z/1 -> ZudX1 q+10/2, ZudX1 q+9/2, ZudX1 q+8/2, ZudX1 q+7/2, ZudX1 q+6/2
  ZudX1 q+10/1 -> Mux/5
  ZudX1 q+6/1 -> Mux/1
  ZudX1 q+7/1 -> Mux/2
  ZudX1 q+8/1 -> Mux/3
  ZudX1 q+9/1 -> Mux/4
  Mux/1 -> ZdX/1

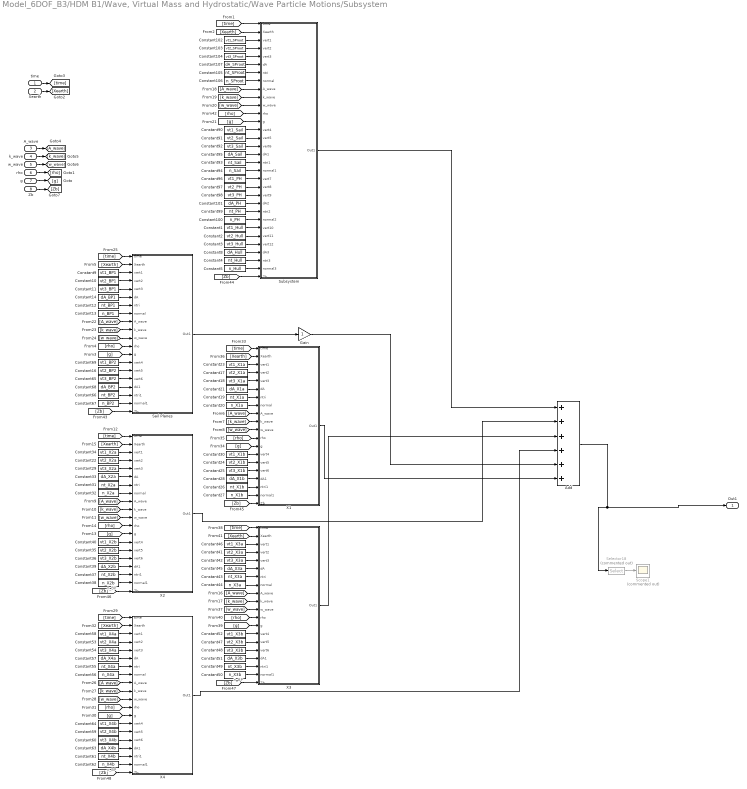
== system Model_6DOF_B3/HDM B1/Wave, Virtual Mass and Hydrostatic/Wave Particle Motions/Subsystem ==
  note: n_BP
  note: n_BP
  note: n_BP
  time : Inport
  Xearth : Inport  Port=2
  A_wave : Inport  Port=3
  k_wave : Inport  Port=4
  w_wave : Inport  Port=5
  rho : Inport  Port=6
  g : Inport  Port=7
  Zb : Inport  Port=8
  Add : Sum  Inputs=6
  Constant1 : Constant  Value=vt1_Hull
  Constant10 : Constant  Value=vt2_BP1
  Constant100 : Constant  Value=n_PH
  Constant101 : Constant  Value=dA_PH
  Constant102 : Constant  Value=vt1_SProot
  Constant103 : Constant  Value=vt2_SProot
  Constant104 : Constant  Value=vt3_SProot
  Constant105 : Constant  Value=nt_SProot
  Constant106 : Constant  Value=n_SProot
  Constant107 : Constant  Value=dA_SProot
  Constant11 : Constant  Value=vt3_BP1
  Constant12 : Constant  Value=nt_BP1
  Constant13 : Constant  Value=n_BP1
  Constant14 : Constant  Value=dA_BP1
  Constant16 : Constant  Value=vt2_BP2
  Constant17 : Constant  Value=vt2_X1a
  Constant18 : Constant  Value=vt3_X1a
  Constant19 : Constant  Value=nt_X1a
  Constant2 : Constant  Value=vt2_Hull
  Constant20 : Constant  Value=n_X1a
  Constant21 : Constant  Value=dA_X1a
  Constant22 : Constant  Value=vt2_X2a
  Constant23 : Constant  Value=vt1_X1a
  Constant24 : Constant  Value=vt2_X1b
  Constant25 : Constant  Value=vt3_X1b
  Constant26 : Constant  Value=nt_X1b
  Constant27 : Constant  Value=n_X1b
  Constant28 : Constant  Value=dA_X1b
  Constant29 : Constant  Value=vt3_X2a
  Constant3 : Constant  Value=vt3_Hull
  Constant30 : Constant  Value=vt1_X1b
  Constant31 : Constant  Value=nt_X2a
  Constant32 : Constant  Value=n_X2a
  Constant33 : Constant  Value=dA_X2a
  Constant34 : Constant  Value=vt1_X2a
  Constant35 : Constant  Value=vt2_X2b
  Constant36 : Constant  Value=vt3_X2b
  Constant37 : Constant  Value=nt_X2b
  Constant38 : Constant  Value=n_X2b
  Constant39 : Constant  Value=dA_X2b
  Constant4 : Constant  Value=nt_Hull
  Constant40 : Constant  Value=vt1_X2b
  Constant41 : Constant  Value=vt2_X3a
  Constant42 : Constant  Value=vt3_X3a
  Constant43 : Constant  Value=nt_X3a
  Constant44 : Constant  Value=n_X3a
  Constant45 : Constant  Value=dA_X3a
  Constant46 : Constant  Value=vt1_X3a
  Constant47 : Constant  Value=vt2_X3b
  Constant48 : Constant  Value=vt3_X3b
  Constant49 : Constant  Value=nt_X3b
  Constant5 : Constant  Value=n_Hull
  Constant50 : Constant  Value=n_X3b
  Constant51 : Constant  Value=dA_X3b
  Constant52 : Constant  Value=vt1_X3b
  Constant53 : Constant  Value=vt2_X4a
  Constant54 : Constant  Value=vt3_X4a
  Constant55 : Constant  Value=nt_X4a
  Constant56 : Constant  Value=n_X4a
  Constant57 : Constant  Value=dA_X4a
  Constant58 : Constant  Value=vt1_X4a
  Constant59 : Constant  Value=vt2_X4b
  Constant60 : Constant  Value=vt3_X4b
  Constant61 : Constant  Value=nt_X4b
  Constant62 : Constant  Value=n_X4b
  Constant63 : Constant  Value=dA_X4b
  Constant64 : Constant  Value=vt1_X4b
  Constant65 : Constant  Value=vt3_BP2
  Constant66 : Constant  Value=nt_BP2
  Constant67 : Constant  Value=n_BP2
  Constant68 : Constant  Value=dA_BP2
  Constant69 : Constant  Value=vt1_BP2
  Constant8 : Constant  Value=dA_Hull
  Constant9 : Constant  Value=vt1_BP1
  Constant90 : Constant  Value=vt1_Sail
  Constant91 : Constant  Value=vt2_Sail
  Constant92 : Constant  Value=vt3_Sail
  Constant93 : Constant  Value=nt_Sail
  Constant94 : Constant  Value=n_Sail
  Constant95 : Constant  Value=dA_Sail
  Constant96 : Constant  Value=vt1_PH
  Constant97 : Constant  Value=vt2_PH
  Constant98 : Constant  Value=vt3_PH
  Constant99 : Constant  Value=nt_PH
  Gain : Gain
  Sail Planes : Subsystem
  Scope1 : Scope  Commented=on
  Selector18 : Selector  Commented=on  InputPortWidth=6  IndexOptions=Index vector (dialog)  Indices=2  OutputSizes=1
  Subsystem : Subsystem
  X1 : Subsystem
  X2 : Subsystem
  X3 : Subsystem
  X4 : Subsystem
  Out1 : Outport
  wires:
  Selector18/1 -> Scope1/1
  Zb/1 -> [Zb]
  [A_wave] -> X3/9(A_wave)
  Constant5/1 -> Subsystem/31(normal3)
  Constant58/1 -> X4/3(vert1)
  Constant42/1 -> X3/5(vert3)
  [g] -> Sail Planes/13(g)
  Constant3/1 -> Subsystem/28(vert12)
  Constant103/1 -> Subsystem/4(vert2)
  Add/1 -> Out1/1, Selector18/1
  [A_wave] -> Subsystem/9(A_wave)
  Constant50/1 -> X3/19(normal1)
  Constant10/1 -> Sail Planes/4(vert2)
  [time] -> X4/1(time)
  [k_wave] -> X4/10(k_wave)
  X2/1(Out1) -> Add/2
  Constant38/1 -> X2/19(normal1)
  X1/1(Out1) -> Add/6
  Constant54/1 -> X4/5(vert3)
  Constant66/1 -> Sail Planes/18(ntri1)
  Constant2/1 -> Subsystem/27(vert11)
  Constant97/1 -> Subsystem/21(vert8)
  Constant64/1 -> X4/14(vert4)
  [Xearth] -> X4/2(Xearth)
  Constant29/1 -> X2/5(vert3)
  Constant36/1 -> X2/16(vert6)
  Constant96/1 -> Subsystem/20(vert7)
  Constant90/1 -> Subsystem/14(vert4)
  Constant21/1 -> X1/6(dA)
  [w_wave] -> X2/11(w_wave)
  Constant31/1 -> X2/7(ntri)
  Constant1/1 -> Subsystem/26(vert10)
  [time] -> X1/1(time)
  Constant91/1 -> Subsystem/15(vert5)
  [rho] -> X1/12(rho)
  [time] -> X2/1(time)
  Constant30/1 -> X1/14(vert4)
  Constant92/1 -> Subsystem/16(vert6)
  Constant100/1 -> Subsystem/25(normal2)
  [w_wave] -> X1/11(w_wave)
  [g] -> X3/13(g)
  X4/1(Out1) -> Add/4
  Constant20/1 -> X1/8(normal)
  Constant12/1 -> Sail Planes/7(ntri)
  Constant24/1 -> X1/15(vert5)
  Constant56/1 -> X4/8(normal)
  Constant26/1 -> X1/18(ntri1)
  [A_wave] -> Sail Planes/9(A_wave)
  Constant62/1 -> X4/19(normal1)
  Constant9/1 -> Sail Planes/3(vert1)
  Constant23/1 -> X1/3(vert1)
  Constant46/1 -> X3/3(vert1)
  Constant68/1 -> Sail Planes/17(dA1)
  [k_wave] -> Sail Planes/10(k_wave)
  Constant17/1 -> X1/4(vert2)
  [A_wave] -> X2/9(A_wave)
  [k_wave] -> X3/10(k_wave)
  Constant43/1 -> X3/7(ntri)
  Constant69/1 -> Sail Planes/14(vert4)
  Constant13/1 -> Sail Planes/8(normal)
  Constant104/1 -> Subsystem/5(vert3)
  Constant65/1 -> Sail Planes/16(vert6)
  [Zb] -> Subsystem/32(Zb)
  Constant67/1 -> Sail Planes/19(normal1)
  Constant25/1 -> X1/16(vert6)
  [Xearth] -> X3/2(Xearth)
  X3/1(Out1) -> Add/3
  Constant14/1 -> Sail Planes/6(dA)
  Sail Planes/1(Out1) -> Gain/1
  Constant52/1 -> X3/14(vert4)
  Constant51/1 -> X3/17(dA1)
  Constant59/1 -> X4/15(vert5)
  Constant4/1 -> Subsystem/30(ntri3)
  [rho] -> Sail Planes/12(rho)
  [time] -> Sail Planes/1(time)
  [Xearth] -> X2/2(Xearth)
  [w_wave] -> Sail Planes/11(w_wave)
  Constant53/1 -> X4/4(vert2)
  [k_wave] -> X1/10(k_wave)
  Constant44/1 -> X3/8(normal)
  [w_wave] -> X4/11(w_wave)
  Constant47/1 -> X3/15(vert5)
  Constant32/1 -> X2/8(normal)
  Constant39/1 -> X2/17(dA1)
  Constant35/1 -> X2/15(vert5)
  [g] -> X1/13(g)
  Constant18/1 -> X1/5(vert3)
  Constant40/1 -> X2/14(vert4)
  Constant45/1 -> X3/6(dA)
  Constant55/1 -> X4/7(ntri)
  Gain/1 -> Add/5
  [rho] -> X3/12(rho)
  Constant27/1 -> X1/19(normal1)
  [rho] -> X2/12(rho)
  [Xearth] -> Sail Planes/2(Xearth)
  Constant49/1 -> X3/18(ntri1)
  Constant22/1 -> X2/4(vert2)
  [k_wave] -> X2/10(k_wave)
  Constant41/1 -> X3/4(vert2)
  [A_wave] -> X1/9(A_wave)
  Constant63/1 -> X4/17(dA1)
  Constant34/1 -> X2/3(vert1)
  Constant11/1 -> Sail Planes/5(vert3)
  [g] -> X4/13(g)
  Constant105/1 -> Subsystem/7(ntri)
  Constant107/1 -> Subsystem/6(dA)
  [Xearth] -> Subsystem/2(Xearth)
  Constant106/1 -> Subsystem/8(normal)
  Constant102/1 -> Subsystem/3(vert1)
  [g] -> Subsystem/13(g)
  Constant19/1 -> X1/7(ntri)
  [k_wave] -> Subsystem/10(k_wave)
  Constant60/1 -> X4/16(vert6)
  [rho] -> Subsystem/12(rho)
  Constant48/1 -> X3/16(vert6)
  [time] -> Subsystem/1(time)
  [rho] -> X4/12(rho)
  Constant33/1 -> X2/6(dA)
  [A_wave] -> X4/9(A_wave)
  Constant95/1 -> Subsystem/17(dA1)
  Constant8/1 -> Subsystem/29(dA3)
  [w_wave] -> X3/11(w_wave)
  Constant28/1 -> X1/17(dA1)
  [g] -> X2/13(g)
  Constant93/1 -> Subsystem/18(ntri1)
  [w_wave] -> Subsystem/11(w_wave)
  [Xearth] -> X1/2(Xearth)
  [time] -> X3/1(time)
  [Zb] -> Sail Planes/20(Zb)
  Constant37/1 -> X2/18(ntri1)
  Constant99/1 -> Subsystem/24(ntri2)
  Constant98/1 -> Subsystem/22(vert9)
  [Zb] -> X2/20(Zb)
  Subsystem/1(Out1) -> Add/1
  [Zb] -> X1/20(Zb)
  Constant16/1 -> Sail Planes/15(vert5)
  Constant101/1 -> Subsystem/23(dA2)
  [Zb] -> X3/20(Zb)
  [Zb] -> X4/20(Zb)
  Constant57/1 -> X4/6(dA)
  Constant61/1 -> X4/18(ntri1)
  Constant94/1 -> Subsystem/19(normal1)
  g/1 -> [g]
  rho/1 -> [rho]
  w_wave/1 -> [w_wave]
  k_wave/1 -> [k_wave]
  A_wave/1 -> [A_wave]
  Xearth/1 -> [Xearth]
  time/1 -> [time]
